simulink model "MPCtest"  (R2021b)
settings: Solver=VariableStepAuto  StartTime=0.0  StopTime=30  RelTol=1e-3  EnableMultiTasking=on
libraries: simulink x1
settings Model: Creator=yinch  LastModifiedBy=Jing
settings SolverCC: AlgebraicLoopSolver=TrustRegion
settings DataIOCC: SaveFormat=Array  ReturnWorkspaceOutputs=off
settings OptimizationCC: LifeSpan=inf
settings DebuggingCC: SFUnexpectedBacktrackingDiag=warning  SFNoUnconditionalDefaultTransitionDiag=warning  SFMachineParentedDataDiag=warning  ArithmeticOperatorsInVariantConditions=warning
settings SFSimCC: SimUseLocalCustomCode=off  CustomCodeUndefinedFunction=UseInterfaceOnly
settings RTWCC: RTWUseLocalCustomCode=off
settings CodeAppCC: StateflowObjectComments=on
settings GRTTargetCC: TargetLangStandard=C89/C90 (ANSI)
settings ConfigComp: CovMetricSettings=dw  CovSaveCumulativeToWorkspaceVar=on  CovSaveSingleToWorkspaceVar=on  CovExternalEMLEnable=off

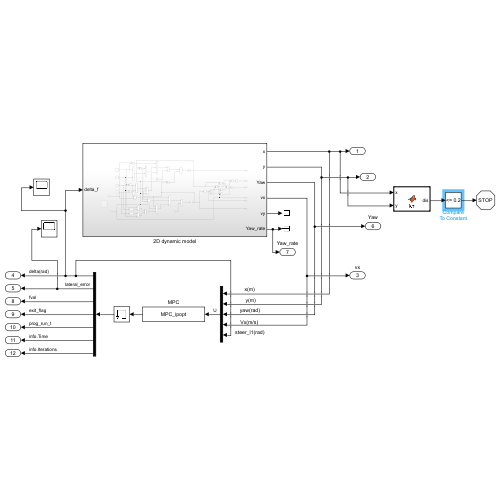
[thumbnail: Simulink's stored preview of the top-level diagram]
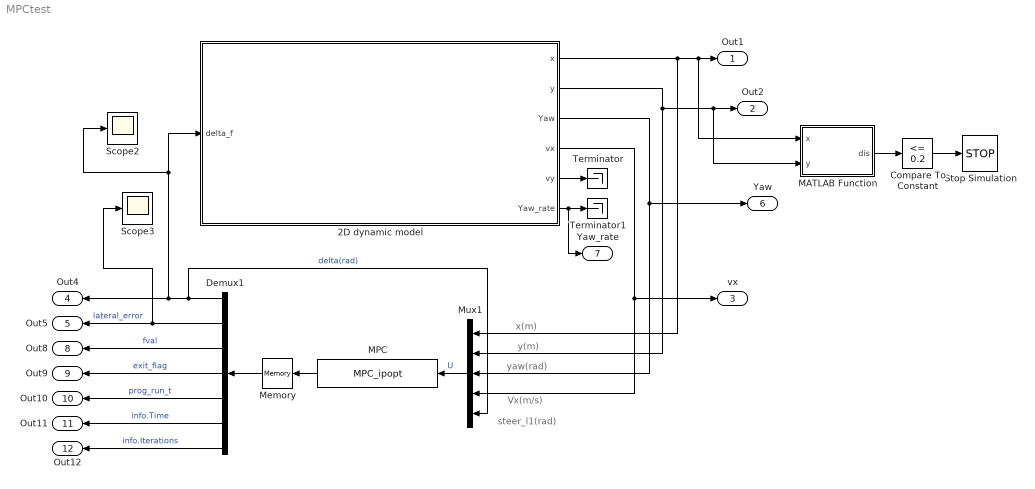
== system MPCtest ==
  note: x(m)
  note: y(m)
  note: yaw(rad)
  note: Vx(m/s)
  note: steer_l1(rad)
  2D dynamic model : Subsystem
  Compare To Constant : simulink/Logic and Bit Operations/Compare To Constant  relop=<=  const=0.2  OutDataTypeStr=boolean
  Demux1 : Demux  Outputs=7
  MATLAB Function : MATLAB Function  TreatAsAtomicUnit=on
  MPC : S-Function  FunctionName=MPC_ipopt  SFunctionDeploymentMode=off  EnableBusSupport=off
  Memory : Memory
  Mux1 : Mux  Inputs=5
  Scope2 : Scope
  Scope3 : Scope
  Stop Simulation : Stop
  Terminator : Terminator
  Terminator1 : Terminator
  Out1 : Outport  VectorParamsAs1DForOutWhenUnconnected=off
  Out2 : Outport  Port=2  VectorParamsAs1DForOutWhenUnconnected=off
  vx : Outport  Port=3  VectorParamsAs1DForOutWhenUnconnected=off
  Out4 : Outport  Port=4  VectorParamsAs1DForOutWhenUnconnected=off
  Out5 : Outport  Port=5  VectorParamsAs1DForOutWhenUnconnected=off
  Yaw : Outport  Port=6  VectorParamsAs1DForOutWhenUnconnected=off
  Yaw_rate : Outport  Port=7  VectorParamsAs1DForOutWhenUnconnected=off
  Out8 : Outport  Port=8  VectorParamsAs1DForOutWhenUnconnected=off
  Out9 : Outport  Port=9  VectorParamsAs1DForOutWhenUnconnected=off
  Out10 : Outport  Port=10  VectorParamsAs1DForOutWhenUnconnected=off
  Out11 : Outport  Port=11  VectorParamsAs1DForOutWhenUnconnected=off
  Out12 : Outport  Port=12  VectorParamsAs1DForOutWhenUnconnected=off
  wires:
  Mux1/1 -> MPC/1  "U"
  MPC/1 -> Memory/1
  Demux1/1 -> Mux1/5, Scope2/1, 2D dynamic model/1(delta_f), Out4/1  "delta(rad)"
  Demux1/2 -> Scope3/1, Out5/1  "lateral_error"
  Memory/1 -> Demux1/1
  Demux1/3 -> Out8/1  "fval"
  Demux1/4 -> Out9/1  "exit_flag"
  Demux1/5 -> Out10/1  "prog_run_t"
  Demux1/6 -> Out11/1  "info.Time"
  Demux1/7 -> Out12/1  "info.Iterations"
  2D dynamic model/1(x) -> Out1/1, MATLAB Function/1(x), Mux1/1
  2D dynamic model/2(y) -> Mux1/2, Out2/1, MATLAB Function/2(y)
  2D dynamic model/3(Yaw) -> Mux1/3, Yaw/1
  2D dynamic model/4(vx) -> vx/1, Mux1/4
  2D dynamic model/5(vy) -> Terminator/1
  2D dynamic model/6(Yaw_rate) -> Yaw_rate/1, Terminator1/1
  MATLAB Function/1(dis) -> Compare To Constant/1
  Compare To Constant/1 -> Stop Simulation/1

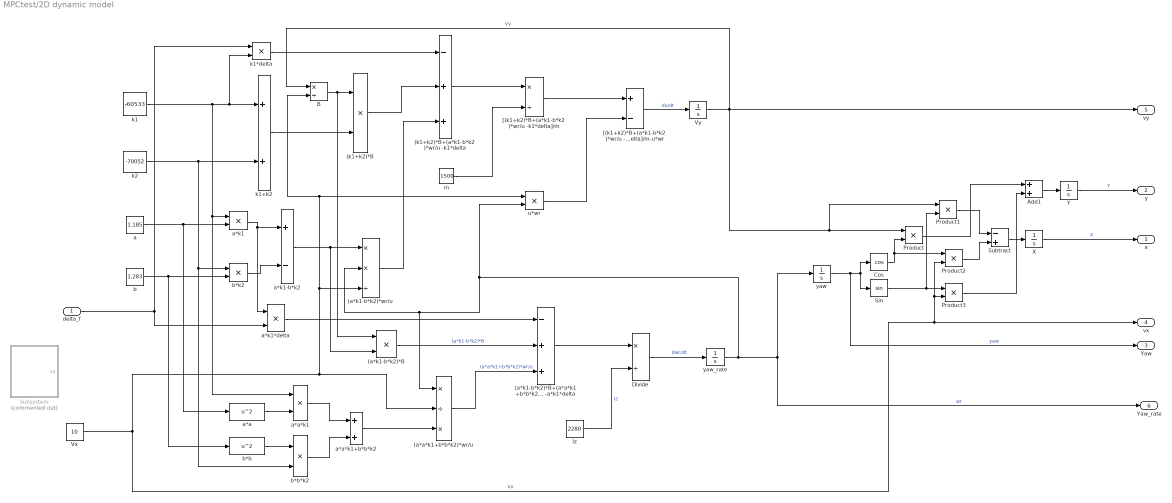
== system MPCtest/2D dynamic model ==
  delta_f : Inport
  (a*a*k1+b*b*k2)*wr/u : Product  Inputs=*/*
  (a*k1-b*k2)*B : Product
  (a*k1-b*k2)*B+(a*a*k1+b*b*k2)*wr/u -a*k1*delta : Sum  Inputs=-++
  (a*k1-b*k2)*wr/u : Product  Inputs=**/
  (k1+k2)*B : Product
  (k1+k2)*B+(a*k1-b*k2)*wr/u -k1*delta : Sum  Inputs=-++
  Add1 : Sum
  B : Product  Inputs=*/
  Cos : Trigonometry  Operator=cos
  Divide : Product  Inputs=*/
  Iz : Constant  Value=2280
  Product{,1..3} (4 alike) : Product
  Sin : Trigonometry
  Subsystem : Subsystem  Commented=on
  Subtract : Sum  Inputs=-+
  Vx : Constant  Value=10
  Vy : Integrator
  X : Integrator
  Y : Integrator
  "[(k1+k2)*B+(a*k1-b*k2)*wr/u -k1*delta]/m" : Product  Inputs=*/
  "[(k1+k2)*B+(a*k1-b*k2)*wr/u -k1*delta]/m-u*wr" : Sum  Inputs=+-
  a : Constant  Value=1.185
  a*a : Fcn  Expr=u^2
  a*a*k1 : Product
  a*a*k1+b*b*k2 : Sum
  a*k1 : Product
  a*k1*delta : Product
  a*k1-b*k2 : Sum  Inputs=+-
  b : Constant  Value=1.283
  b*b : Fcn  Expr=u^2
  b*b*k2 : Product
  b*k2 : Product
  k1 : Constant  Value=-60533
  k1*delta : Product
  k1+k2 : Sum
  k2 : Constant  Value=-70052
  m : Constant  Value=1500
  u*wr : Product
  yaw : Integrator
  yaw_rate : Integrator
  x : Outport  VectorParamsAs1DForOutWhenUnconnected=off
  y : Outport  Port=2  VectorParamsAs1DForOutWhenUnconnected=off
  Yaw : Outport  Port=3  VectorParamsAs1DForOutWhenUnconnected=off
  vx : Outport  Port=4  VectorParamsAs1DForOutWhenUnconnected=off
  vy : Outport  Port=5  VectorParamsAs1DForOutWhenUnconnected=off
  Yaw_rate : Outport  Port=6  VectorParamsAs1DForOutWhenUnconnected=off
  wires:
  (a*a*k1+b*b*k2)*wr/u/1 -> (a*k1-b*k2)*B+(a*a*k1+b*b*k2)*wr/u -a*k1*delta/3  "(a*a*k1+b*b*k2)*wr/u"
  b/1 -> b*k2/2, b*b/1
  (a*k1-b*k2)*B+(a*a*k1+b*b*k2)*wr/u -a*k1*delta/1 -> Divide/1
  k1+k2/1 -> (k1+k2)*B/2
  yaw/1 -> Yaw/1, Cos/1, Sin/1  "yaw"
  k1/1 -> k1*delta/2, k1+k2/1, a*a*k1/1, a*k1/1
  k2/1 -> k1+k2/2, b*b*k2/2, b*k2/1
  b*b/1 -> b*b*k2/1
  Product2/1 -> Subtract/2
  B/1 -> (a*k1-b*k2)*B/1, (k1+k2)*B/1
  Add1/1 -> Y/1
  Sin/1 -> Product3/1, Product1/2
  "[(k1+k2)*B+(a*k1-b*k2)*wr/u -k1*delta]/m"/1 -> "[(k1+k2)*B+(a*k1-b*k2)*wr/u -k1*delta]/m-u*wr"/1
  yaw_rate/1 -> (a*k1-b*k2)*wr/u/2, (a*a*k1+b*b*k2)*wr/u/1, u*wr/2, yaw/1, Yaw_rate/1  "wr"
  a/1 -> a*k1/2, a*a/1
  Product/1 -> Add1/1
  a*k1-b*k2/1 -> (a*k1-b*k2)*B/2, (a*k1-b*k2)*wr/u/1
  Product3/1 -> Add1/2
  b*b*k2/1 -> a*a*k1+b*b*k2/2
  Vy/1 -> vy/1, Product/1, Product1/1, B/1  "Vy"
  a*a*k1/1 -> a*a*k1+b*b*k2/1
  "[(k1+k2)*B+(a*k1-b*k2)*wr/u -k1*delta]/m-u*wr"/1 -> Vy/1  "dv/dt"
  u*wr/1 -> "[(k1+k2)*B+(a*k1-b*k2)*wr/u -k1*delta]/m-u*wr"/2
  (k1+k2)*B+(a*k1-b*k2)*wr/u -k1*delta/1 -> "[(k1+k2)*B+(a*k1-b*k2)*wr/u -k1*delta]/m"/1
  a*k1/1 -> a*k1*delta/1, a*k1-b*k2/1
  a*a*k1+b*b*k2/1 -> (a*a*k1+b*b*k2)*wr/u/3
  Iz/1 -> Divide/2  "Iz"
  (a*k1-b*k2)*B/1 -> (a*k1-b*k2)*B+(a*a*k1+b*b*k2)*wr/u -a*k1*delta/2  "(a*k1-b*k2)*B"
  (a*k1-b*k2)*wr/u/1 -> (k1+k2)*B+(a*k1-b*k2)*wr/u -k1*delta/3
  Vx/1 -> B/2, u*wr/1, (a*k1-b*k2)*wr/u/3, (a*a*k1+b*b*k2)*wr/u/2, vx/1, Product3/2, Product2/2  "Vx"
  delta_f/1 -> a*k1*delta/2, k1*delta/1
  a*a/1 -> a*a*k1/2
  Y/1 -> y/1  "Y"
  (k1+k2)*B/1 -> (k1+k2)*B+(a*k1-b*k2)*wr/u -k1*delta/2
  Cos/1 -> Product2/1, Product/2
  a*k1*delta/1 -> (a*k1-b*k2)*B+(a*a*k1+b*b*k2)*wr/u -a*k1*delta/1
  b*k2/1 -> a*k1-b*k2/2
  k1*delta/1 -> (k1+k2)*B+(a*k1-b*k2)*wr/u -k1*delta/1
  m/1 -> "[(k1+k2)*B+(a*k1-b*k2)*wr/u -k1*delta]/m"/2
  Divide/1 -> yaw_rate/1  "dwr/dt"
  Subtract/1 -> X/1
  Product1/1 -> Subtract/1
  X/1 -> x/1  "X"

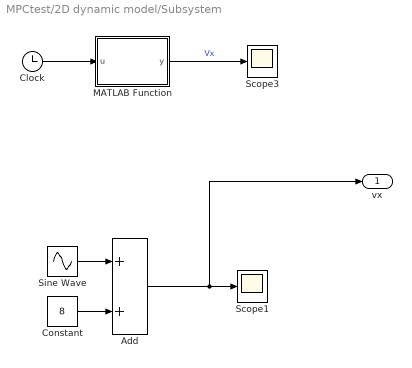
== system MPCtest/2D dynamic model/Subsystem ==
  Add : Sum
  Clock : Clock
  Constant : Constant  Value=8
  MATLAB Function : MATLAB Function  TreatAsAtomicUnit=on
  Scope1 : Scope
  Scope3 : Scope
  Sine Wave : Sin  Amplitude=5  Frequency=0.05*pi  SampleTime=0.1
  vx : Outport
  wires:
  MATLAB Function/1(y) -> Scope3/1  "Vx"
  Sine Wave/1 -> Add/1
  Clock/1 -> MATLAB Function/1(u)
  Add/1 -> vx/1, Scope1/1
  Constant/1 -> Add/2

== matlab function MPCtest/2D dynamic model/Subsystem/MATLAB Function ==
  data: u input; y output
function y = fcn(u)

if u <= 25
    y = 5+0.2*u;
else
    y = 10;
end

== matlab function MPCtest/MATLAB Function ==
  data: x input; dis output; y input
function dis = fcn(x, y)

x0 = -100;
y0 = -100;
dis = ((x-x0)^2 + (y-y0)^2)^0.5;
